simulink model "model_refrigeration_test"  (R2023a)
settings: Solver=VariableStepAuto  StartTime=0.0  StopTime=300  RelTol=1e-3  AbsTol=1e-3
PreLoadFcn:
  | x_init = 0.19;
libraries: fl_lib x68, nesl_utility x14, SimscapeFluids_lib x5, slpidlib x1
(part 2 of 2)

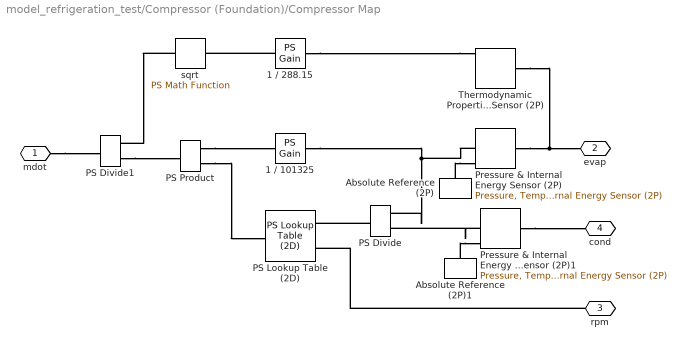
== system model_refrigeration_test/Compressor (Foundation)/Compressor Map ==
  1 / 101325 : fl_lib/Physical Signals/Functions/PS Gain  gain=1 / 101325 1/Pa
  1 / 288.15 : fl_lib/Physical Signals/Functions/PS Gain  gain=1 / 288.15 1/K
  Absolute Reference (2P) : fl_lib/Two-Phase Fluid/Elements/Absolute Reference (2P)
  Absolute Reference (2P)1 : fl_lib/Two-Phase Fluid/Elements/Absolute Reference (2P)
  PS Divide : fl_lib/Physical Signals/Functions/PS Divide
  PS Divide1 : fl_lib/Physical Signals/Functions/PS Divide
  PS Lookup Table (2D) : fl_lib/Physical Signals/Lookup Tables/PS Lookup Table (2D)  x1=[0; 1; 4.28795213348131; 7.57590426696263; 10.8638564004439; 14.1518085339253] Pa/Pa  x2=[0, 1800, 3600] rpm  f=|  interp_method=simscape.enum.interpolation.linear  extrap_method=simscape.enum.extrapolation.nearest
      | [
      | 0, 0, 0;
      | 0, 0.0136946156177912, 0.0273892312355827;
      | 0, 0.0102709617133435, 0.0205419234266869;
      | 0, 0.00684730780889566, 0.0136946156177912;
      | 0, 0.00342365390444783, 0.00684730780889563;
      | 0, 0, 0] * 1.09 kg/s
  PS Product : fl_lib/Physical Signals/Functions/PS Product
  Pressure & Internal Energy Sensor (2P) : fl_lib/Two-Phase Fluid/Sensors/Pressure, Temperature & Internal Energy Sensor (2P)  reference=foundation.enum.MeasurementReference.difference  pressure=true  pressure_spec=foundation.enum.PressureMeasementSpec.Absolute  temperature=false  internal_energy=true
      settings: InternalSimscapePortConfiguration="{\"Bottom\":[{\"id\":\"U\",\"label\":\"U\",\"type\":\"output\"}],\"Left\":[{\"id\":\"A\",\"label\":\"A\",\"type\":\"foundation.two_phase_fluid.two_phase_fluid\"}],\"Right\":[{\"id\":\"B\",\"label\":\"B\",\"type\":\"foundation.two_phase_fluid.two_phase_fluid\"},{\"id\":\"P\",\"label\":\"P\",\"type\":\"output\"}],\"Top\":[]}"
  Pressure & Internal Energy Sensor (2P)1 : fl_lib/Two-Phase Fluid/Sensors/Pressure, Temperature & Internal Energy Sensor (2P)  reference=foundation.enum.MeasurementReference.difference  pressure=true  pressure_spec=foundation.enum.PressureMeasementSpec.Absolute  temperature=false  internal_energy=true
      settings: InternalSimscapePortConfiguration="{\"Bottom\":[{\"id\":\"U\",\"label\":\"U\",\"type\":\"output\"}],\"Left\":[{\"id\":\"A\",\"label\":\"A\",\"type\":\"foundation.two_phase_fluid.two_phase_fluid\"}],\"Right\":[{\"id\":\"B\",\"label\":\"B\",\"type\":\"foundation.two_phase_fluid.two_phase_fluid\"},{\"id\":\"P\",\"label\":\"P\",\"type\":\"output\"}],\"Top\":[]}"
  Thermodynamic Properties Sensor (2P) : fl_lib/Two-Phase Fluid/Sensors/Thermodynamic Properties Sensor (2P)  temperature=true  enthalpy=true  density=false  specific_volume=true  entropy=true
      settings: InternalSimscapePortConfiguration="{\"Bottom\":[{\"id\":\"V\",\"label\":\"v\",\"type\":\"output\"},{\"id\":\"S\",\"label\":\"s\",\"type\":\"output\"}],\"Left\":[{\"id\":\"A\",\"label\":\"A\",\"type\":\"foundation.two_phase_fluid.two_phase_fluid\"}],\"Right\":[{\"id\":\"T\",\"label\":\"T\",\"type\":\"output\"},{\"id\":\"H\",\"label\":\"h\",\"type\":\"output\"}],\"Top\":[]}"
  sqrt : fl_lib/Physical Signals/Functions/PS Math Function  fcn_choice=foundation.enum.math_function.sqrt  v=1
  mdot : PMIOPort  Side=Left
  evap : PMIOPort  Port=2  Side=Right
  rpm : PMIOPort  Port=3  Side=Right
  cond : PMIOPort  Port=4  Side=Right
  connections:
  Absolute Reference (2P)1/LConn1 -- Pressure & Internal Energy Sensor (2P)1/RConn1
  Pressure & Internal Energy Sensor (2P)1/LConn1 -- cond/RConn1
  Absolute Reference (2P)/LConn1 -- Pressure & Internal Energy Sensor (2P)/RConn1
  Pressure & Internal Energy Sensor (2P)/LConn1 -- Thermodynamic Properties Sensor (2P)/LConn1 -- evap/RConn1
  Pressure & Internal Energy Sensor (2P)/RConn2 -- 1 / 101325/LConn1 -- PS Divide/LConn2
  Pressure & Internal Energy Sensor (2P)1/RConn2 -- PS Divide/LConn1
  rpm/RConn1 -- PS Lookup Table (2D)/LConn2
  PS Divide/RConn1 -- PS Lookup Table (2D)/LConn1
  1 / 288.15/LConn1 -- Thermodynamic Properties Sensor (2P)/RConn1
  PS Product/LConn1 -- 1 / 101325/RConn1
  PS Product/LConn2 -- PS Lookup Table (2D)/RConn1
  PS Divide1/LConn1 -- PS Product/RConn1
  1 / 288.15/RConn1 -- sqrt/LConn1
  sqrt/RConn1 -- PS Divide1/LConn2
  mdot/RConn1 -- PS Divide1/RConn1
